simulink model "sensorTask"  (R2015b)
settings: configuration reference "Run_on_Hardware_Configuration" (kept outside this file)
libraries: embdlinuxlib x1, quadLibrary x1
settings Model: DataDictionary=quadCopterDD.sldd  SimulationMode=external  ExtModeEnableFloating=off  ExtModeTrigDuration=100  Creator=Nik Descher  LastModifiedBy=Nik Descher
settings ConfigSetRef: DDName=quadCopterDD.sldd

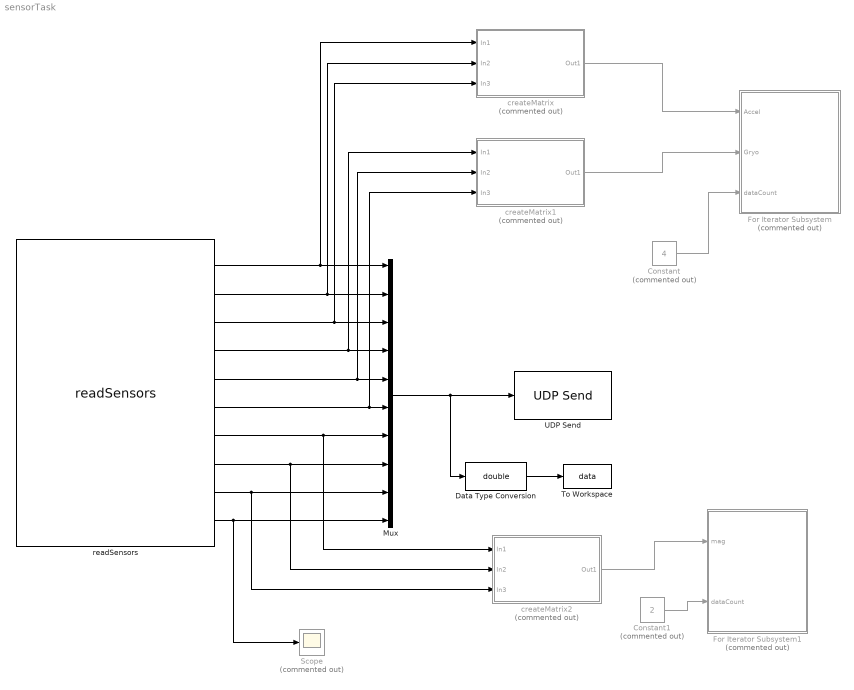
== system sensorTask ==
  Constant : Constant  Commented=on  Value=4
  Constant1 : Constant  Commented=on  Value=2
  Data Type Conversion : DataTypeConversion  OutDataTypeStr=double
  For Iterator Subsystem : Subsystem  Commented=on  TreatAsAtomicUnit=on
  For Iterator Subsystem1 : Subsystem  Commented=on  TreatAsAtomicUnit=on
  Mux : Mux  Inputs=10
  Scope : Scope  Commented=on
  To Workspace : ToWorkspace  VariableName=data  SaveFormat=Structure With Time  SampleTime=-1
  UDP Send : embdlinuxlib/UDP Send  remoteURL='127.0.0.1'  remotePort=25000  localURL='255.255.255.255'  localPortSource=Automatically determine  localPort=-1  sampletime=-1  blockPlatform=Raspberry Pi  separateLengthPort=0
  createMatrix : Subsystem  Commented=on
  createMatrix1 : Subsystem  Commented=on
  createMatrix2 : Subsystem  Commented=on
  readSensors : quadLibrary/readSensors
  wires:
  readSensors/1 -> createMatrix/1(In1), Mux/1
  createMatrix/1(Out1) -> For Iterator Subsystem/1(Accel)
  createMatrix1/1(Out1) -> For Iterator Subsystem/2(Gryo)
  readSensors/6 -> createMatrix1/3(In3), Mux/6
  readSensors/5 -> createMatrix1/2(In2), Mux/5
  readSensors/8 -> createMatrix2/2(In2), Mux/8
  readSensors/9 -> createMatrix2/3(In3), Mux/9
  readSensors/7 -> createMatrix2/1(In1), Mux/7
  readSensors/3 -> createMatrix/3(In3), Mux/3
  readSensors/4 -> createMatrix1/1(In1), Mux/4
  readSensors/2 -> createMatrix/2(In2), Mux/2
  Mux/1 -> Data Type Conversion/1, UDP Send/1
  Constant/1 -> For Iterator Subsystem/3(dataCount)
  Constant1/1 -> For Iterator Subsystem1/2(dataCount)
  createMatrix2/1(Out1) -> For Iterator Subsystem1/1(mag)
  readSensors/10 -> Mux/10, Scope/1
  Data Type Conversion/1 -> To Workspace/1

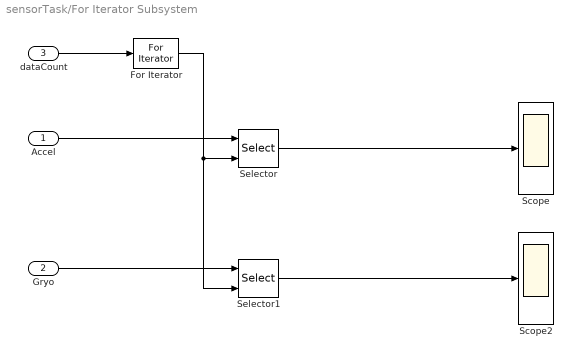
== system sensorTask/For Iterator Subsystem ==
  Accel : Inport
  Gryo : Inport  Port=2
  dataCount : Inport  Port=3
  For Iterator : ForIterator  IterationSource=external
  Scope : Scope
  Scope2 : Scope
  Selector : Selector  NumberOfDimensions=2  InputPortWidth=3  IndexOptions=Index vector (dialog),Index vector (port)  Indices=[1 2 3],1  OutputSizes=1,1
  Selector1 : Selector  NumberOfDimensions=2  InputPortWidth=3  IndexOptions=Index vector (dialog),Index vector (port)  Indices=[1 2 3],1  OutputSizes=1,1
  wires:
  Selector1/1 -> Scope2/1
  Gryo/1 -> Selector1/1
  Selector/1 -> Scope/1
  For Iterator/1 -> Selector/2, Selector1/2
  Accel/1 -> Selector/1
  dataCount/1 -> For Iterator/1

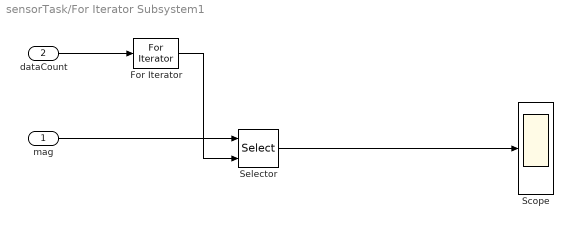
== system sensorTask/For Iterator Subsystem1 ==
  mag : Inport
  dataCount : Inport  Port=2
  For Iterator : ForIterator  IterationSource=external
  Scope : Scope
  Selector : Selector  NumberOfDimensions=2  InputPortWidth=3  IndexOptions=Index vector (dialog),Index vector (port)  Indices=[1 2 3],1  OutputSizes=1,1
  wires:
  dataCount/1 -> For Iterator/1
  mag/1 -> Selector/1
  For Iterator/1 -> Selector/2
  Selector/1 -> Scope/1

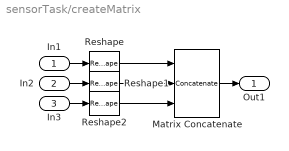
== system sensorTask/createMatrix ==
  In1 : Inport
  In2 : Inport  Port=2
  In3 : Inport  Port=3
  Matrix Concatenate : Concatenate  NumInputs=3  Mode=Multidimensional array
  Reshape : Reshape  OutputDimensionality=Row vector (2-D)
  Reshape1 : Reshape  OutputDimensionality=Row vector (2-D)
  Reshape2 : Reshape  OutputDimensionality=Row vector (2-D)
  Out1 : Outport
  wires:
  Reshape/1 -> Matrix Concatenate/1
  Reshape2/1 -> Matrix Concatenate/3
  Reshape1/1 -> Matrix Concatenate/2
  In3/1 -> Reshape2/1
  In2/1 -> Reshape1/1
  Matrix Concatenate/1 -> Out1/1
  In1/1 -> Reshape/1

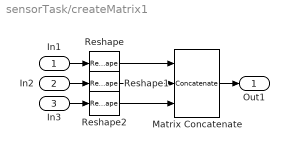
== system sensorTask/createMatrix1 ==
  In1 : Inport
  In2 : Inport  Port=2
  In3 : Inport  Port=3
  Matrix Concatenate : Concatenate  NumInputs=3  Mode=Multidimensional array
  Reshape : Reshape  OutputDimensionality=Row vector (2-D)
  Reshape1 : Reshape  OutputDimensionality=Row vector (2-D)
  Reshape2 : Reshape  OutputDimensionality=Row vector (2-D)
  Out1 : Outport
  wires:
  In1/1 -> Reshape/1
  Matrix Concatenate/1 -> Out1/1
  In2/1 -> Reshape1/1
  In3/1 -> Reshape2/1
  Reshape1/1 -> Matrix Concatenate/2
  Reshape2/1 -> Matrix Concatenate/3
  Reshape/1 -> Matrix Concatenate/1

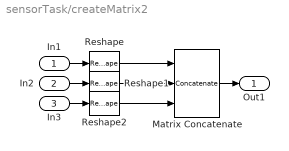
== system sensorTask/createMatrix2 ==
  In1 : Inport
  In2 : Inport  Port=2
  In3 : Inport  Port=3
  Matrix Concatenate : Concatenate  NumInputs=3  Mode=Multidimensional array
  Reshape : Reshape  OutputDimensionality=Row vector (2-D)
  Reshape1 : Reshape  OutputDimensionality=Row vector (2-D)
  Reshape2 : Reshape  OutputDimensionality=Row vector (2-D)
  Out1 : Outport
  wires:
  Reshape/1 -> Matrix Concatenate/1
  Reshape2/1 -> Matrix Concatenate/3
  Reshape1/1 -> Matrix Concatenate/2
  In3/1 -> Reshape2/1
  In2/1 -> Reshape1/1
  Matrix Concatenate/1 -> Out1/1
  In1/1 -> Reshape/1
